simulink model "audioSignalGen"  (R2020b)
settings: Solver=FixedStepDiscrete  StartTime=0.0  StopTime=inf  RelTol=1e-3
PreLoadFcn:
  | paramSignalGen
values from neighbouring files (symbols this model uses):
  freqTable = [20 50 100 200 300 400 500 600 700 800 900 1000 1200,     1400 1600 1800 2000 2400 2800 3200 3500 4000 4500 5000,     5500 6000 6500 7000 7500 8000 8500 9000]    [paramSignalGen.m]
libraries: hdlsllib x15, simulink x2
settings Model: DataTypeOverride=Off  PacingRate=0.890000  Creator=amatsumo  LastModifiedBy=amatsumo
settings DataIOCC: SaveOutput=off  SaveTime=off
settings OptimizationCC: BlockReduction=off  ConditionallyExecuteInputs=off  DefaultParameterBehavior=Inlined
settings DebuggingCC: AlgebraicLoopMsg=error  SingleTaskRateTransMsg=error  ParameterOverflowMsg=warning  StrictBusMsg=ErrorOnBusTreatedAsVector  ArithmeticOperatorsInVariantConditions=warning
settings HardwareCC: ProdBitPerPointer=32  ProdBitPerSizeT=32  ProdBitPerPtrDiffT=32  ProdLargestAtomicFloat=None  ProdIntDivRoundTo=Undefined  ProdEndianess=Unspecified  ProdWordSize=32  ProdHWDeviceType=ASIC/FPGA->ASIC/FPGA  ProdEqTarget=off
settings SFSimCC: SimUseLocalCustomCode=off  CustomCodeUndefinedFunction=UseInterfaceOnly
settings RTWCC: RTWUseLocalCustomCode=off
settings CodeAppCC: StateflowObjectComments=on
settings GRTTargetCC: TargetLangStandard=C89/C90 (ANSI)

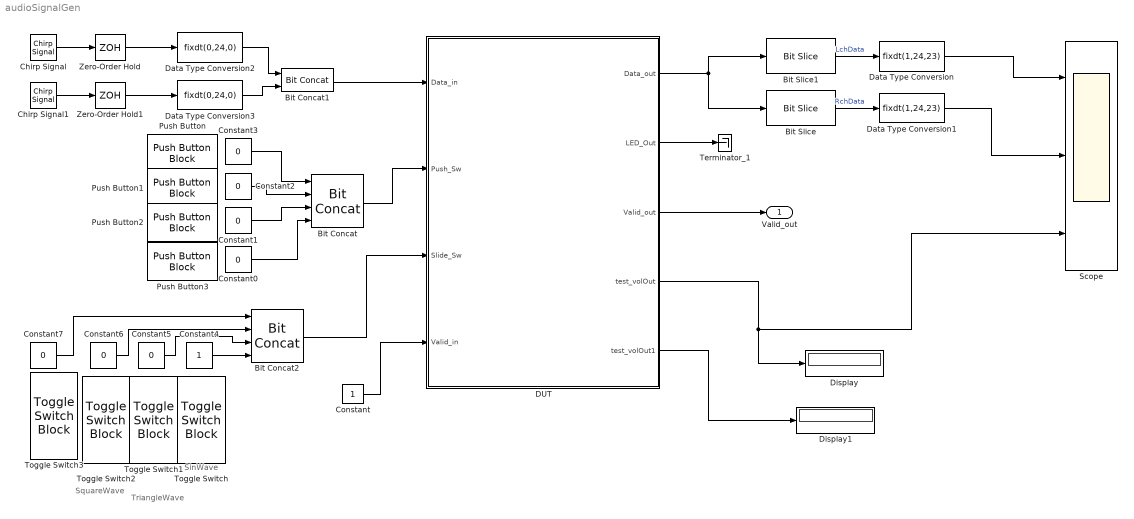
== system audioSignalGen ==
  note: SinWave
  note: TriangleWave
  note: SquareWave
  Bit Concat : hdlsllib/Logic and Bit Operations/Bit Concat  numInputs=4
  Bit Concat1 : hdlsllib/Logic and Bit Operations/Bit Concat  numInputs=2
  Bit Concat2 : hdlsllib/Logic and Bit Operations/Bit Concat  numInputs=4
  Bit Slice : hdlsllib/Logic and Bit Operations/Bit Slice  lidx=23  ridx=0
      settings: SourceProductBaseCode=SL
  Bit Slice1 : hdlsllib/Logic and Bit Operations/Bit Slice  lidx=47  ridx=24
      settings: SourceProductBaseCode=SL
  Chirp Signal : simulink/Sources/Chirp Signal  f1=10  T=10  f2=1000
  Chirp Signal1 : simulink/Sources/Chirp Signal  f1=1000  T=10  f2=10
  Constant : Constant  OutDataTypeStr=boolean  SampleTime=-1
  Constant{0..3,5..7} (7 alike) : Constant  Value=0  OutDataTypeStr=boolean  SampleTime=-1
  Constant4 : Constant  OutDataTypeStr=boolean  SampleTime=-1
  DUT : Subsystem  TreatAsAtomicUnit=on
  Data Type Conversion : DataTypeConversion  OutDataTypeStr=fixdt(1,24,23)  ConvertRealWorld=Stored Integer (SI)  LockScale=on
  Data Type Conversion1 : DataTypeConversion  OutDataTypeStr=fixdt(1,24,23)  ConvertRealWorld=Stored Integer (SI)  LockScale=on
  Data Type Conversion2 : DataTypeConversion  OutDataTypeStr=fixdt(0,24,0)  ConvertRealWorld=Stored Integer (SI)  LockScale=on
  Data Type Conversion3 : DataTypeConversion  OutDataTypeStr=fixdt(0,24,0)  ConvertRealWorld=Stored Integer (SI)  LockScale=on
  Display : Display
  Display1 : Display
  Push Button : PushButtonBlock  ButtonText=KEY3
  Push Button1 : PushButtonBlock  ButtonText=KEY2
  Push Button2 : PushButtonBlock  ButtonText=KEY1
  Push Button3 : PushButtonBlock  ButtonText=KEY0
  Scope : Scope  NumInputPorts=3
  Terminator_1 : Terminator
  Toggle Switch{,1..3} (4 alike) : ToggleSwitchBlock
      settings: Values={{'Off', 'On'}, [0 1]}
  Zero-Order Hold : ZeroOrderHold  SampleTime=1/48000
  Zero-Order Hold1 : ZeroOrderHold  SampleTime=1/48000
  Valid_out : Outport  VectorParamsAs1DForOutWhenUnconnected=off
  wires:
  DUT/1(Data_out) -> Bit Slice/1, Bit Slice1/1
  Bit Concat1/1 -> DUT/1(Data_in)
  DUT/3(Valid_out) -> Valid_out/1
  Constant/1 -> DUT/4(Valid_in)
  Constant3/1 -> Bit Concat/1
  Bit Concat/1 -> DUT/2(Push_Sw)
  Constant2/1 -> Bit Concat/2
  Constant1/1 -> Bit Concat/3
  Constant0/1 -> Bit Concat/4
  DUT/4(test_volOut) -> Display/1, Scope/3
  Bit Slice1/1 -> Data Type Conversion/1  "LchData"
  Bit Slice/1 -> Data Type Conversion1/1  "RchData"
  Data Type Conversion/1 -> Scope/1
  Data Type Conversion1/1 -> Scope/2
  Data Type Conversion2/1 -> Bit Concat1/1
  Data Type Conversion3/1 -> Bit Concat1/2
  Chirp Signal/1 -> Zero-Order Hold/1
  Zero-Order Hold/1 -> Data Type Conversion2/1
  Chirp Signal1/1 -> Zero-Order Hold1/1
  Zero-Order Hold1/1 -> Data Type Conversion3/1
  Constant4/1 -> Bit Concat2/4
  Constant5/1 -> Bit Concat2/3
  Constant6/1 -> Bit Concat2/2
  Constant7/1 -> Bit Concat2/1
  Bit Concat2/1 -> DUT/3(Slide_Sw)
  DUT/5(test_volOut1) -> Display1/1
  DUT/2(LED_Out) -> Terminator_1/1

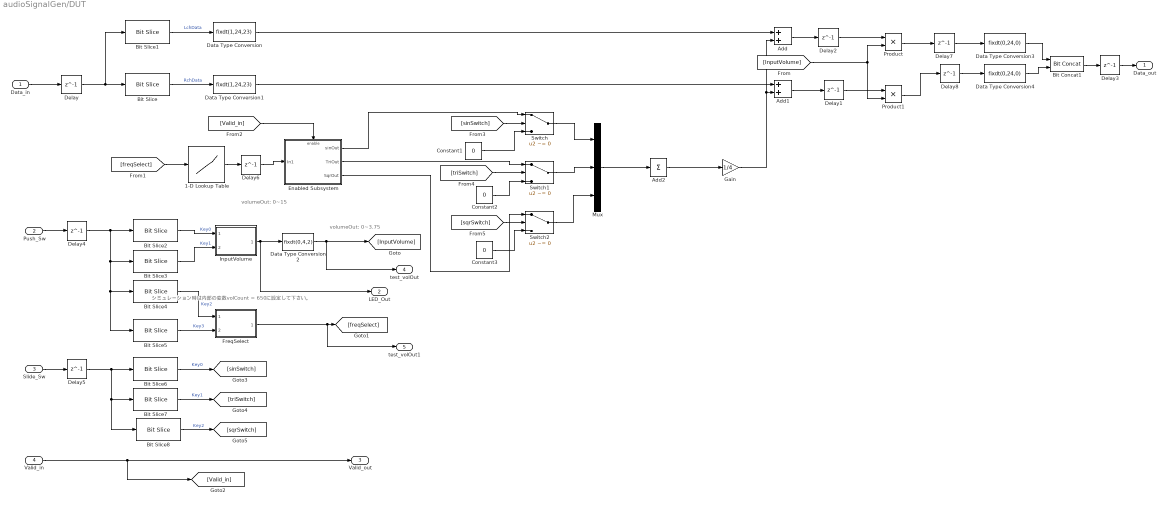
== system audioSignalGen/DUT ==
  note: volumeOut: 0~15
  note: シミュレーション時は内部の変数volCount = 650に設定して下さい。
  note: volumeOut: 0~3.75
  Data_in : Inport  OutDataTypeStr=fixdt(0,48,0)
  Push_Sw : Inport  Port=2
  Slide_Sw : Inport  Port=3
  Valid_in : Inport  Port=4  OutDataTypeStr=boolean
  1-D Lookup Table : Lookup_n-D  NumberOfTableDimensions=1  LookupTableObject=''  BreakpointsForDimension1=[0:31]  BreakpointsForDimension1FirstPoint=10  BreakpointsForDimension2FirstPoint=10  BreakpointsForDimension1Spacing=12  BreakpointsForDimension2Spacing=12  IndexSearchMethod=Evenly spaced points  Table=freqTable  TableDataTypeStr=fixdt(0,16,0)  InterpMethod=Flat  DiagnosticForOutOfRangeInput=Error  InternalRulePriority=Speed  OutDataTypeStr=fixdt(0,16,0)  RndMeth=Simplest  InputSameDT=on
  Add : Sum  OutDataTypeStr=Inherit: Same as first input
  Add1 : Sum  OutDataTypeStr=Inherit: Same as first input
  Add2 : Sum  Inputs=+
  Bit Concat1 : hdlsllib/Logic and Bit Operations/Bit Concat  numInputs=2
  Bit Slice : hdlsllib/Logic and Bit Operations/Bit Slice  lidx=23  ridx=0
      settings: SourceProductBaseCode=SL
  Bit Slice1 : hdlsllib/Logic and Bit Operations/Bit Slice  lidx=47  ridx=24
      settings: SourceProductBaseCode=SL
  Bit Slice2 : hdlsllib/Logic and Bit Operations/Bit Slice  lidx=0  ridx=0
      settings: SourceProductBaseCode=SL
  Bit Slice3 : hdlsllib/Logic and Bit Operations/Bit Slice  lidx=1  ridx=1
      settings: SourceProductBaseCode=SL
  Bit Slice4 : hdlsllib/Logic and Bit Operations/Bit Slice  lidx=2  ridx=2
      settings: SourceProductBaseCode=SL
  Bit Slice5 : hdlsllib/Logic and Bit Operations/Bit Slice  lidx=3  ridx=3
      settings: SourceProductBaseCode=SL
  Bit Slice6 : hdlsllib/Logic and Bit Operations/Bit Slice  lidx=0  ridx=0
      settings: SourceProductBaseCode=SL
  Bit Slice7 : hdlsllib/Logic and Bit Operations/Bit Slice  lidx=1  ridx=1
      settings: SourceProductBaseCode=SL
  Bit Slice8 : hdlsllib/Logic and Bit Operations/Bit Slice  lidx=2  ridx=2
      settings: SourceProductBaseCode=SL
  Constant1 : Constant  Value=0  OutDataTypeStr=Inherit: Inherit via back propagation  SampleTime=-1
  Constant2 : Constant  Value=0  OutDataTypeStr=Inherit: Inherit via back propagation  SampleTime=-1
  Constant3 : Constant  Value=0  OutDataTypeStr=Inherit: Inherit via back propagation  SampleTime=-1
  Data Type Conversion : DataTypeConversion  OutDataTypeStr=fixdt(1,24,23)  ConvertRealWorld=Stored Integer (SI)
  Data Type Conversion1 : DataTypeConversion  OutDataTypeStr=fixdt(1,24,23)  ConvertRealWorld=Stored Integer (SI)
  Data Type Conversion2 : DataTypeConversion  OutDataTypeStr=fixdt(0,4,2)  ConvertRealWorld=Stored Integer (SI)
  Data Type Conversion3 : DataTypeConversion  OutDataTypeStr=fixdt(0,24,0)  ConvertRealWorld=Stored Integer (SI)  LockScale=on
  Data Type Conversion4 : DataTypeConversion  OutDataTypeStr=fixdt(0,24,0)  ConvertRealWorld=Stored Integer (SI)  LockScale=on
  Delay{,1..8} (9 alike) : Delay  DelayLength=1
  Enabled Subsystem : Subsystem  TreatAsAtomicUnit=on
  FreqSelect : MATLAB Function  TreatAsAtomicUnit=on
  Gain : Gain  Gain=1/4  ParamDataTypeStr=fixdt(0,4)  SaturateOnIntegerOverflow=on  OutDataTypeStr=Inherit: Same as input
  InputVolume : MATLAB Function  TreatAsAtomicUnit=on
  Mux : Mux  Inputs=3
  Product : Product  SaturateOnIntegerOverflow=on  OutDataTypeStr=Inherit: Same as first input
  Product1 : Product  SaturateOnIntegerOverflow=on  OutDataTypeStr=Inherit: Same as first input
  Switch : Switch  Criteria=u2 ~= 0
  Switch1 : Switch  Criteria=u2 ~= 0
  Switch2 : Switch  Criteria=u2 ~= 0
  Data_out : Outport  OutDataTypeStr=fixdt(0,48,0)  VectorParamsAs1DForOutWhenUnconnected=off
  LED_Out : Outport  Port=2  VectorParamsAs1DForOutWhenUnconnected=off
  Valid_out : Outport  Port=3  OutDataTypeStr=boolean  VectorParamsAs1DForOutWhenUnconnected=off
  test_volOut : Outport  Port=4  VectorParamsAs1DForOutWhenUnconnected=off
  test_volOut1 : Outport  Port=5  VectorParamsAs1DForOutWhenUnconnected=off
  wires:
  Valid_in/1 -> [Valid_in], Valid_out/1
  Delay/1 -> Bit Slice1/1, Bit Slice/1
  Bit Slice1/1 -> Data Type Conversion/1  "LchData"
  Bit Slice/1 -> Data Type Conversion1/1  "RchData"
  Delay4/1 -> Bit Slice5/1, Bit Slice4/1, Bit Slice3/1, Bit Slice2/1
  Bit Slice2/1 -> InputVolume/1(pushSwUp)  "Key0"
  InputVolume/1(volumeOut) -> Data Type Conversion2/1, LED_Out/1
  Bit Slice3/1 -> InputVolume/2(pushSwDown)  "Key1"
  Bit Slice4/1 -> FreqSelect/1(pushSwUp)  "Key2"
  Bit Slice5/1 -> FreqSelect/2(pushSwDown)  "Key3"
  Data Type Conversion2/1 -> [InputVolume], test_volOut/1
  Data Type Conversion/1 -> Add/1
  Data Type Conversion1/1 -> Add1/1
  FreqSelect/1(volumeOut) -> test_volOut1/1, [freqSelect]
  [Valid_in] -> Enabled Subsystem/Enable
  [freqSelect] -> 1-D Lookup Table/1
  Enabled Subsystem/1(sinOut) -> Switch/1
  Delay5/1 -> Bit Slice8/1, Bit Slice7/1, Bit Slice6/1
  Bit Slice6/1 -> [sinSwitch]  "Key0"
  Bit Slice7/1 -> [triSwitch]  "Key1"
  Bit Slice8/1 -> [sqrSwitch]  "Key2"
  [sinSwitch] -> Switch/2
  Constant1/1 -> Switch/3
  [triSwitch] -> Switch1/2
  Enabled Subsystem/2(TriOut) -> Switch1/1
  Constant2/1 -> Switch1/3
  Enabled Subsystem/3(SqrOut) -> Switch2/1
  [sqrSwitch] -> Switch2/2
  Constant3/1 -> Switch2/3
  Switch/1 -> Mux/1
  Switch1/1 -> Mux/2
  Switch2/1 -> Mux/3
  Mux/1 -> Add2/1
  Add/1 -> Delay2/1
  [InputVolume] -> Product1/2, Product/2
  Add1/1 -> Delay1/1
  Data Type Conversion4/1 -> Bit Concat1/2
  Data Type Conversion3/1 -> Bit Concat1/1
  Bit Concat1/1 -> Delay3/1
  Product/1 -> Delay7/1
  Product1/1 -> Delay8/1
  Gain/1 -> Add/2, Add1/2
  Delay2/1 -> Product/1
  Delay1/1 -> Product1/1
  Delay3/1 -> Data_out/1
  Add2/1 -> Gain/1
  Data_in/1 -> Delay/1
  Push_Sw/1 -> Delay4/1
  Slide_Sw/1 -> Delay5/1
  1-D Lookup Table/1 -> Delay6/1
  Delay6/1 -> Enabled Subsystem/1(In1)
  Delay7/1 -> Data Type Conversion3/1
  Delay8/1 -> Data Type Conversion4/1

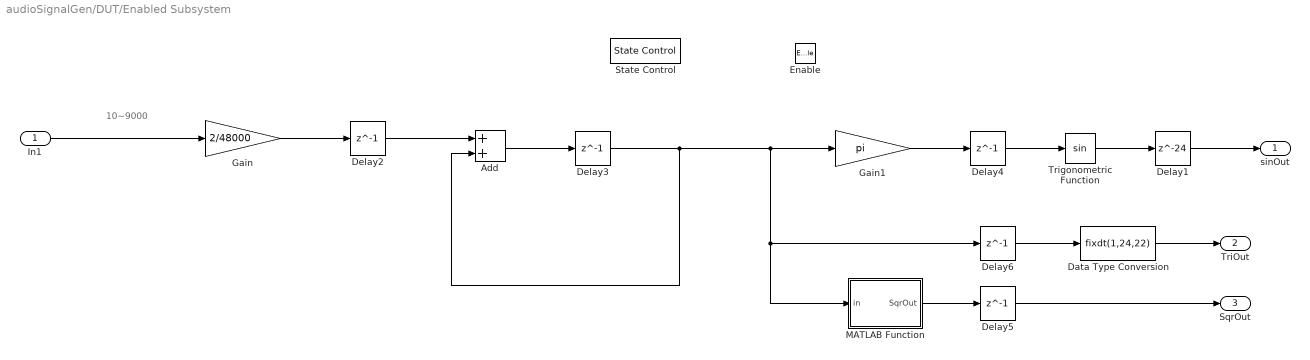
== system audioSignalGen/DUT/Enabled Subsystem ==
  note: 10~9000
  In1 : Inport
  Enable : EnablePort
  Add : Sum  OutMin=-1  OutMax=0.99  OutDataTypeStr=fixdt(1,18,17)
  Data Type Conversion : DataTypeConversion  OutDataTypeStr=fixdt(1,24,22)
  Delay1 : Delay  DelayLength=24
  Delay{2..6} (5 alike) : Delay  DelayLength=1
  Gain : Gain  Gain=2/48000  ParamDataTypeStr=fixdt(0,16)  OutMin=10/48000  OutMax=9000/48000  OutDataTypeStr=fixdt(0,18,20)
  Gain1 : Gain  Gain=pi  ParamDataTypeStr=fixdt(0,16,13)  OutMin=-2*pi  OutMax=2*pi*0.999  OutDataTypeStr=fixdt(1,24,20)
  MATLAB Function : MATLAB Function  TreatAsAtomicUnit=on
  State Control : StateControl  StateControl=Synchronous
  Trigonometric Function : Trigonometry  ApproximationMethod=CORDIC  NumberOfIterations=23
  sinOut : Outport  InitialOutput=0
  TriOut : Outport  Port=2  InitialOutput=0
  SqrOut : Outport  Port=3  InitialOutput=0
  wires:
  Trigonometric Function/1 -> Delay1/1
  Gain/1 -> Delay2/1
  Add/1 -> Delay3/1
  Delay3/1 -> MATLAB Function/1(in), Delay6/1, Gain1/1, Add/2
  Gain1/1 -> Delay4/1
  In1/1 -> Gain/1
  Delay2/1 -> Add/1
  Delay4/1 -> Trigonometric Function/1
  Delay6/1 -> Data Type Conversion/1
  Delay5/1 -> SqrOut/1
  Delay1/1 -> sinOut/1
  MATLAB Function/1(SqrOut) -> Delay5/1
  Data Type Conversion/1 -> TriOut/1

== matlab function audioSignalGen/DUT/InputVolume ==
  settings: fimath=hdlfimath;
  data: pushSwUp input; volumeOut output; pushSwDown input
function volumeOut = fcn(pushSwUp, pushSwDown)
%#codegen
if coder.target('HDL')
    volCount = 65000;
else
    % simulation
    volCount = 650;   % for Test
end

persistent countUpBuf valueStoredUp countDownBuf valueStoredDown volumeBuf
if isempty(countUpBuf)
    countUpBuf = fi(0, 0, 16, 0, 'OverflowAction', 'Saturate');
    valueStoredUp = fi(0,0,1,0);
    countDownBuf = fi(0, 0, 16, 0, 'OverflowAction', 'Saturate');
    valueStoredDown = fi(0,0,1,0);
    volumeBuf = fi(6, 0, 4, 0, 'OverflowAction', 'Wrap');     % Volume 0~15
end

% Up count
if pushSwUp > valueStoredUp   % pushSwUp=1, valueStoredUp=0
    countUpBuf(:) = countUpBuf + 1;
else
    countUpBuf(:) = 0;
    valueStoredUp = pushSwUp;
end

% Down count
if pushSwDown > valueStoredDown    % pushSwDown=1, valueStoredDown=0
    countDownBuf(:) = countDownBuf + 1;
else
    countDownBuf(:) = 0;
    valueStoredDown = pushSwDown;
end

% Volume Change
if countUpBuf > volCount
    volumeBuf(:) = volumeBuf +1;
    countUpBuf(:) = 0;
    valueStoredUp = pushSwUp;
%     valueStoredUp = true;
end
if countDownBuf > volCount
    volumeBuf(:) = volumeBuf -1;
    countDownBuf(:) = 0;
    valueStoredDown = pushSwDown;
%     valueStoredDown = true;
end
volumeOut = volumeBuf;




% Update

== matlab function audioSignalGen/DUT/Enabled Subsystem/MATLAB Function ==
  data: in input; SqrOut output
function SqrOut = fcn(in)

if in > 0
    SqrOut = fi(0.99, 1, 24, 22);
else
    SqrOut = fi(-1, 1, 24, 22);
end

== matlab function audioSignalGen/DUT/FreqSelect ==
  settings: fimath=hdlfimath;
  data: pushSwUp input; volumeOut output; pushSwDown input
function volumeOut = fcn(pushSwUp, pushSwDown)
%#codegen
if coder.target('HDL')
    volCount = 65000;
else
    % simulation
    volCount = 650;   % for Test
end


persistent countUpBuf valueStoredUp countDownBuf valueStoredDown volumeBuf
if isempty(countUpBuf)
    countUpBuf = fi(0, 0, 16, 0, 'OverflowAction', 'Saturate');
    valueStoredUp = fi(0,0,1,0);
    countDownBuf = fi(0, 0, 16, 0, 'OverflowAction', 'Saturate');
    valueStoredDown = fi(0,0,1,0);
    volumeBuf = fi(10, 0, 5, 0, 'OverflowAction', 'Wrap');     % select 0~31
end

% Up count
if pushSwUp > valueStoredUp   % pushSwUp=1, valueStoredUp=0
    countUpBuf(:) = countUpBuf + 1;
else
    countUpBuf(:) = 0;
    valueStoredUp = pushSwUp;
end

% Down count
if pushSwDown > valueStoredDown    % pushSwDown=1, valueStoredDown=0
    countDownBuf(:) = countDownBuf + 1;
else
    countDownBuf(:) = 0;
    valueStoredDown = pushSwDown;
end

% Volume Change
if countUpBuf > volCount
    volumeBuf(:) = volumeBuf +1;
    countUpBuf(:) = 0;
    valueStoredUp = pushSwUp;
%     valueStoredUp = true;
end
if countDownBuf > volCount
    volumeBuf(:) = volumeBuf -1;
    countDownBuf(:) = 0;
    valueStoredDown = pushSwDown;
%     valueStoredDown = true;
end
volumeOut = volumeBuf;




% Update
